simulink library "X_Plane_Communication_Library"  (R2013a)
settings: Solver=ode45  StartTime=0.0  StopTime=10.0  RelTol=1e-3
libraries: dspnetwork x4, etargetslib x4
settings Model: Creator=Adriano  LastModifiedBy=Adriano

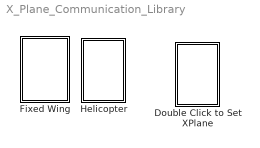
== system X_Plane_Communication_Library ==
  Double Click to Set XPlane : Subsystem
      settings: OpenFcn=selecting_parameters()
  Fixed Wing : Subsystem
  Helicopter : Subsystem

== system X_Plane_Communication_Library/Double Click to Set XPlane ==

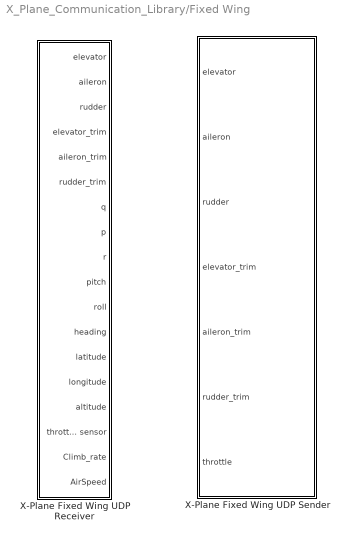
== system X_Plane_Communication_Library/Fixed Wing ==
  X-Plane Fixed Wing UDP Receiver : Subsystem  mask{ip_adress='127.0.0.1', port_number=49004}
      mask prompts: ip_adress "Local IP Adress (default: '127.0.0.1' )"; port_number "Output Port Number (defaut: '49004')"
      mask help: This block is configured to receiver data from a fixed wing aircraft on X-Plane Flight Simulator.
      mask Help: Contact adrianobittar@gmail.com
  X-Plane Fixed Wing UDP Sender : Subsystem  mask{ip_adress='127.0.0.1', port_number=49000}
      mask prompts: ip_adress "Local IP Adress (default: '127.0.0.1' )"; port_number "Output Port Number (defaut: '49000')"
      mask help: This block is configured to send data to a fixed wing aircraft on X-Plane Flight Simulator.
      mask Help: Contact adrianobittar@gmail.com

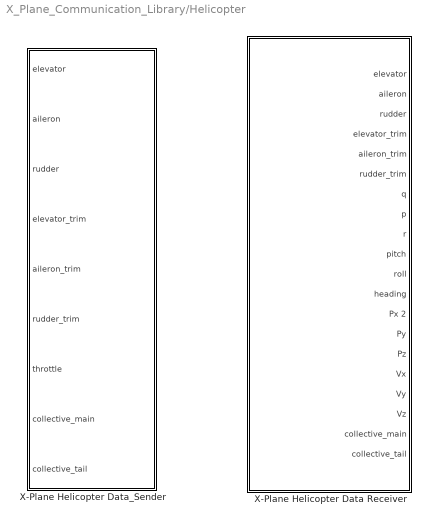
== system X_Plane_Communication_Library/Helicopter ==
  X-Plane Helicopter Data Receiver : Subsystem  AncestorBlock=DU2SRI_Heli_Sim/X-Plane Communication Blockset /X-Plane Data Receiver  mask{ip_adress='127.0.0.1', port_number=49004}
      mask prompts: ip_adress "Local IP Adress (default: '127.0.0.1')"; port_number "Input Port Number (default: '49004')"
      mask help: This block is configured to receive data to an helicopter aircraft on X-Plane Flight Simulator.
      mask Help: Contact adrianobittar@gmail.com
  X-Plane Helicopter Data_Sender : Subsystem  AncestorBlock=DU2SRI_Heli_Sim/X-Plane Communication Blockset /X-Plane Data_Sender  mask{ip_address='127.0.0.1', port_number=49000, max_col_main=12, min_col_main=0, max_col_tail=5, min_col_tail=-5}
      mask prompts: ip_address "Local IP Address (default: '127.0.0.1' )"; port_number "Output Port Number (defaut: '49000')"; max_col_main "Max Angle For Collective Main"; min_col_main "Min Angle For Collective Main"; max_col_tail "Max Angle For Collective Tail"; min_col_tail "Min Angle For Collective Tail"
      mask help: This block is configured to send data to an helicopter aircraft on X-Plane Flight Simulator.
      mask Help: contact adrianobittar@gmail.com

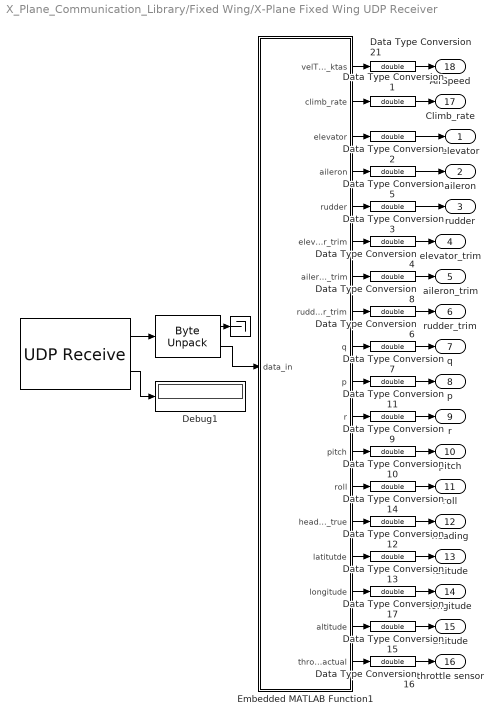
== system X_Plane_Communication_Library/Fixed Wing/X-Plane Fixed Wing UDP Receiver ==
  " " : Terminator
  "    " : dspnetwork/UDP Receive  localURL='0.0.0.0'  localPort=port_number  remoteURL=ip_adress  remotePort=-1  recvBufferSize=8192  dims=293  signalDatatype=uint8  isVarSize=off  showBlockingTime=on  blockingTime=20  sampletime=0.02  blockPlatform=WINDOWS
  "     " : etargetslib/Byte Unpack  dimensions={5,[9,8]}  datatypes={'uint8','single'}  byteAlign=1
  Data Type Conversion{1..17,21} (18 alike) : DataTypeConversion  OutDataTypeStr=double  SaturateOnIntegerOverflow=on
  "Debug1 " : Display
  Embedded MATLAB Function1 : MATLAB Function  TreatAsAtomicUnit=on
  "elevator " : Outport
  aileron : Outport  Port=2
  rudder : Outport  Port=3
  elevator_trim : Outport  Port=4
  aileron_trim : Outport  Port=5
  rudder_trim : Outport  Port=6
  q : Outport  Port=7
  p : Outport  Port=8
  r : Outport  Port=9
  pitch : Outport  Port=10
  roll : Outport  Port=11
  heading : Outport  Port=12
  latitude : Outport  Port=13
  longitude : Outport  Port=14
  altitude : Outport  Port=15
  throttle sensor : Outport  Port=16
  Climb_rate : Outport  Port=17
  AirSpeed : Outport  Port=18
  wires:
  "     "/2 -> Embedded MATLAB Function1/1(data_in)
  Data Type Conversion9/1 -> r/1
  "    "/1 -> "     "/1
  Data Type Conversion10/1 -> pitch/1
  "    "/2 -> "Debug1 "/1
  "     "/1 -> " "/1
  Embedded MATLAB Function1/1(velTrue_ktas) -> Data Type Conversion21/1
  Embedded MATLAB Function1/18(throttle_actual) -> Data Type Conversion16/1
  Embedded MATLAB Function1/17(altitude) -> Data Type Conversion15/1
  Embedded MATLAB Function1/16(longitude) -> Data Type Conversion17/1
  Embedded MATLAB Function1/15(latitutde) -> Data Type Conversion13/1
  Embedded MATLAB Function1/14(heading_true) -> Data Type Conversion12/1
  Embedded MATLAB Function1/13(roll) -> Data Type Conversion14/1
  Embedded MATLAB Function1/12(pitch) -> Data Type Conversion10/1
  Embedded MATLAB Function1/11(r) -> Data Type Conversion9/1
  Embedded MATLAB Function1/10(p) -> Data Type Conversion11/1
  Embedded MATLAB Function1/9(q) -> Data Type Conversion7/1
  Embedded MATLAB Function1/8(rudder_trim) -> Data Type Conversion6/1
  Embedded MATLAB Function1/7(aileron_trim) -> Data Type Conversion8/1
  Embedded MATLAB Function1/6(elevator_trim) -> Data Type Conversion4/1
  Embedded MATLAB Function1/5(rudder) -> Data Type Conversion3/1
  Embedded MATLAB Function1/4(aileron) -> Data Type Conversion5/1
  Embedded MATLAB Function1/3(elevator) -> Data Type Conversion2/1
  Embedded MATLAB Function1/2(climb_rate) -> Data Type Conversion1/1
  Data Type Conversion21/1 -> AirSpeed/1
  Data Type Conversion1/1 -> Climb_rate/1
  Data Type Conversion2/1 -> "elevator "/1
  Data Type Conversion5/1 -> aileron/1
  Data Type Conversion8/1 -> aileron_trim/1
  Data Type Conversion3/1 -> rudder/1
  Data Type Conversion4/1 -> elevator_trim/1
  Data Type Conversion6/1 -> rudder_trim/1
  Data Type Conversion7/1 -> q/1
  Data Type Conversion12/1 -> heading/1
  Data Type Conversion13/1 -> latitude/1
  Data Type Conversion14/1 -> roll/1
  Data Type Conversion17/1 -> longitude/1
  Data Type Conversion15/1 -> altitude/1
  Data Type Conversion16/1 -> throttle sensor/1
  Data Type Conversion11/1 -> p/1

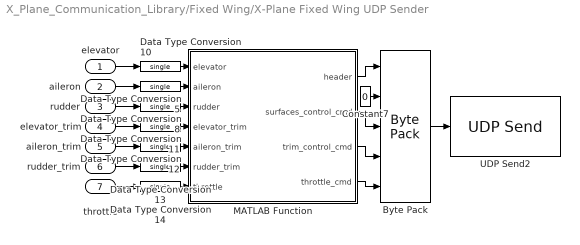
== system X_Plane_Communication_Library/Fixed Wing/X-Plane Fixed Wing UDP Sender ==
  elevator : Inport
  aileron : Inport  Port=2
  rudder : Inport  Port=3
  elevator_trim : Inport  Port=4
  aileron_trim : Inport  Port=5
  rudder_trim : Inport  Port=6
  throttle : Inport  Port=7
  Byte Pack : etargetslib/Byte Pack  datatypes={'single','uint8','single','single','single'}  byteAlign=1
  Constant7 : Constant  Value=0  OutDataTypeStr=uint8
  Data Type Conversion{5,8,10..14} (7 alike) : DataTypeConversion  OutDataTypeStr=single  SaturateOnIntegerOverflow=on
  MATLAB Function : MATLAB Function  TreatAsAtomicUnit=on
  UDP Send2 : dspnetwork/UDP Send  remoteURL=ip_adress  remotePort=port_number  localURL='255.255.255.255'  localPortSource=Automatically determine  localPort=-1  sampletime=-1  blockPlatform=HOST  separateLengthPort=0
  wires:
  rudder/1 -> Data Type Conversion8/1
  Constant7/1 -> Byte Pack/2
  Data Type Conversion8/1 -> MATLAB Function/3(rudder)
  throttle/1 -> Data Type Conversion14/1
  Data Type Conversion10/1 -> MATLAB Function/1(elevator)
  Data Type Conversion11/1 -> MATLAB Function/4(elevator_trim)
  aileron/1 -> Data Type Conversion5/1
  elevator/1 -> Data Type Conversion10/1
  MATLAB Function/4(throttle_cmd) -> Byte Pack/5
  Data Type Conversion5/1 -> MATLAB Function/2(aileron)
  Data Type Conversion14/1 -> MATLAB Function/7(throttle)
  MATLAB Function/3(trim_control_cmd) -> Byte Pack/4
  aileron_trim/1 -> Data Type Conversion12/1
  Data Type Conversion13/1 -> MATLAB Function/6(rudder_trim)
  Data Type Conversion12/1 -> MATLAB Function/5(aileron_trim)
  MATLAB Function/1(header) -> Byte Pack/1
  elevator_trim/1 -> Data Type Conversion11/1
  Byte Pack/1 -> UDP Send2/1
  MATLAB Function/2(surfaces_control_cmd) -> Byte Pack/3
  rudder_trim/1 -> Data Type Conversion13/1

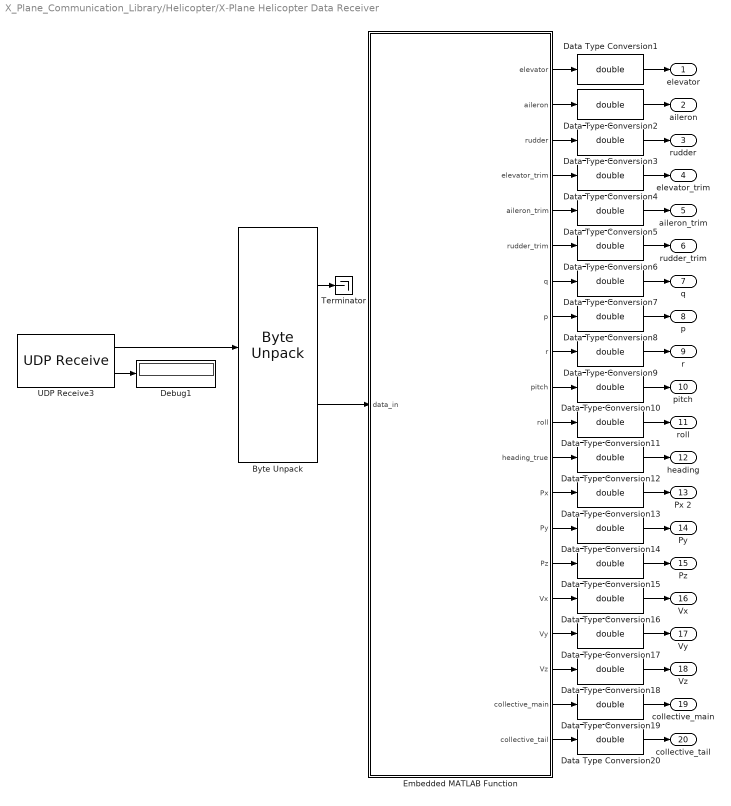
== system X_Plane_Communication_Library/Helicopter/X-Plane Helicopter Data Receiver ==
  Byte Unpack : etargetslib/Byte Unpack  dimensions={5,[9,6]}  datatypes={'uint8','single'}  byteAlign=1
  Data Type Conversion{1..20} (20 alike) : DataTypeConversion  OutDataTypeStr=double  SaturateOnIntegerOverflow=on
  "Debug1 " : Display
  Embedded MATLAB Function : MATLAB Function  TreatAsAtomicUnit=on
  Terminator : Terminator
  UDP Receive3 : dspnetwork/UDP Receive  localURL='0.0.0.0'  localPort=port_number  remoteURL=ip_adress  remotePort=-1  recvBufferSize=8192  dims=221  signalDatatype=uint8  isVarSize=off  showBlockingTime=on  blockingTime=20  sampletime=0  blockPlatform=WINDOWS
  "elevator " : Outport
  aileron : Outport  Port=2
  rudder : Outport  Port=3
  elevator_trim : Outport  Port=4
  aileron_trim : Outport  Port=5
  rudder_trim : Outport  Port=6
  q : Outport  Port=7
  p : Outport  Port=8
  r : Outport  Port=9
  pitch : Outport  Port=10
  roll : Outport  Port=11
  heading : Outport  Port=12
  Px 2 : Outport  Port=13
  Py : Outport  Port=14
  Pz : Outport  Port=15
  Vx : Outport  Port=16
  Vy : Outport  Port=17
  Vz : Outport  Port=18
  collective_main : Outport  Port=19
  collective_tail : Outport  Port=20
  wires:
  Embedded MATLAB Function/10(pitch) -> Data Type Conversion10/1
  Data Type Conversion8/1 -> p/1
  Data Type Conversion13/1 -> Px 2/1
  Data Type Conversion1/1 -> "elevator "/1
  Byte Unpack/1 -> Terminator/1
  UDP Receive3/2 -> "Debug1 "/1
  Data Type Conversion4/1 -> elevator_trim/1
  Embedded MATLAB Function/8(p) -> Data Type Conversion8/1
  Data Type Conversion12/1 -> heading/1
  Embedded MATLAB Function/11(roll) -> Data Type Conversion11/1
  Embedded MATLAB Function/1(elevator) -> Data Type Conversion1/1
  Data Type Conversion10/1 -> pitch/1
  Embedded MATLAB Function/3(rudder) -> Data Type Conversion3/1
  Data Type Conversion2/1 -> aileron/1
  Data Type Conversion6/1 -> rudder_trim/1
  UDP Receive3/1 -> Byte Unpack/1
  Data Type Conversion9/1 -> r/1
  Data Type Conversion11/1 -> roll/1
  Embedded MATLAB Function/7(q) -> Data Type Conversion7/1
  Embedded MATLAB Function/18(Vz) -> Data Type Conversion18/1
  Data Type Conversion18/1 -> Vz/1
  Data Type Conversion5/1 -> aileron_trim/1
  Data Type Conversion15/1 -> Pz/1
  Data Type Conversion19/1 -> collective_main/1
  Embedded MATLAB Function/14(Py) -> Data Type Conversion14/1
  Embedded MATLAB Function/5(aileron_trim) -> Data Type Conversion5/1
  Embedded MATLAB Function/19(collective_main) -> Data Type Conversion19/1
  Embedded MATLAB Function/6(rudder_trim) -> Data Type Conversion6/1
  Embedded MATLAB Function/20(collective_tail) -> Data Type Conversion20/1
  Data Type Conversion16/1 -> Vx/1
  Embedded MATLAB Function/12(heading_true) -> Data Type Conversion12/1
  Embedded MATLAB Function/13(Px) -> Data Type Conversion13/1
  Data Type Conversion17/1 -> Vy/1
  Embedded MATLAB Function/4(elevator_trim) -> Data Type Conversion4/1
  Data Type Conversion14/1 -> Py/1
  Embedded MATLAB Function/17(Vy) -> Data Type Conversion17/1
  Embedded MATLAB Function/2(aileron) -> Data Type Conversion2/1
  Embedded MATLAB Function/16(Vx) -> Data Type Conversion16/1
  Data Type Conversion3/1 -> rudder/1
  Embedded MATLAB Function/15(Pz) -> Data Type Conversion15/1
  Embedded MATLAB Function/9(r) -> Data Type Conversion9/1
  Data Type Conversion7/1 -> q/1
  Data Type Conversion20/1 -> collective_tail/1
  Byte Unpack/2 -> Embedded MATLAB Function/1(data_in)

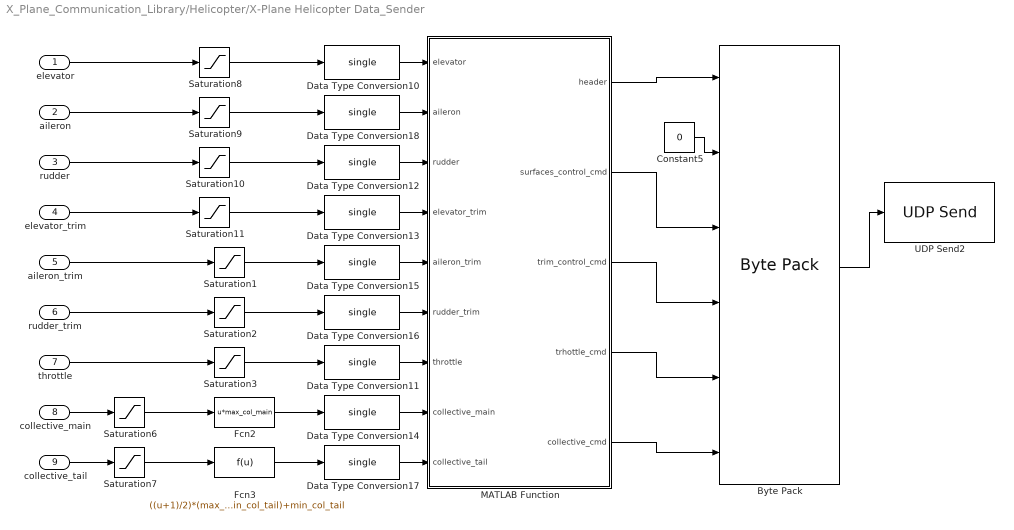
== system X_Plane_Communication_Library/Helicopter/X-Plane Helicopter Data_Sender ==
  elevator : Inport
  aileron : Inport  Port=2
  rudder : Inport  Port=3
  elevator_trim : Inport  Port=4
  aileron_trim : Inport  Port=5
  rudder_trim : Inport  Port=6
  throttle : Inport  Port=7
  collective_main : Inport  Port=8
  collective_tail : Inport  Port=9
  Byte Pack : etargetslib/Byte Pack  datatypes={'single','uint8','single','single','single','single'}  byteAlign=1
  Constant5 : Constant  Value=0  OutDataTypeStr=uint8
  Data Type Conversion{10..18} (9 alike) : DataTypeConversion  OutDataTypeStr=single  SaturateOnIntegerOverflow=on
  Fcn2 : Fcn  Expr=u*max_col_main
  Fcn3 : Fcn  Expr=((u+1)/2)*(max_col_tail-min_col_tail)+min_col_tail
  MATLAB Function : MATLAB Function  TreatAsAtomicUnit=on
  Saturation{1..3,6..11} (9 alike) : Saturate  UpperLimit=+1  LowerLimit=-1
  UDP Send2 : dspnetwork/UDP Send  remoteURL=ip_address  remotePort=port_number  localURL='255.255.255.255'  localPortSource=Automatically determine  localPort=-1  sampletime=-1  blockPlatform=HOST  separateLengthPort=0
  wires:
  Saturation8/1 -> Data Type Conversion10/1
  Data Type Conversion18/1 -> MATLAB Function/2(aileron)
  Constant5/1 -> Byte Pack/2
  MATLAB Function/5(collective_cmd) -> Byte Pack/6
  MATLAB Function/4(trhottle_cmd) -> Byte Pack/5
  MATLAB Function/3(trim_control_cmd) -> Byte Pack/4
  MATLAB Function/2(surfaces_control_cmd) -> Byte Pack/3
  MATLAB Function/1(header) -> Byte Pack/1
  Byte Pack/1 -> UDP Send2/1
  Data Type Conversion17/1 -> MATLAB Function/9(collective_tail)
  Data Type Conversion14/1 -> MATLAB Function/8(collective_main)
  Data Type Conversion11/1 -> MATLAB Function/7(throttle)
  Data Type Conversion16/1 -> MATLAB Function/6(rudder_trim)
  Data Type Conversion15/1 -> MATLAB Function/5(aileron_trim)
  Data Type Conversion13/1 -> MATLAB Function/4(elevator_trim)
  Data Type Conversion12/1 -> MATLAB Function/3(rudder)
  Data Type Conversion10/1 -> MATLAB Function/1(elevator)
  Saturation10/1 -> Data Type Conversion12/1
  Saturation11/1 -> Data Type Conversion13/1
  Saturation9/1 -> Data Type Conversion18/1
  Saturation7/1 -> Fcn3/1
  Saturation6/1 -> Fcn2/1
  collective_main/1 -> Saturation6/1
  collective_tail/1 -> Saturation7/1
  Saturation3/1 -> Data Type Conversion11/1
  elevator_trim/1 -> Saturation11/1
  Saturation1/1 -> Data Type Conversion15/1
  aileron/1 -> Saturation9/1
  Saturation2/1 -> Data Type Conversion16/1
  elevator/1 -> Saturation8/1
  Fcn2/1 -> Data Type Conversion14/1
  rudder/1 -> Saturation10/1
  aileron_trim/1 -> Saturation1/1
  rudder_trim/1 -> Saturation2/1
  throttle/1 -> Saturation3/1
  Fcn3/1 -> Data Type Conversion17/1

== matlab function X_Plane_Communication_Library/Fixed Wing/X-Plane Fixed Wing UDP Receiver/Embedded MATLAB Function1 ==
  data: velTrue_ktas output; climb_rate output; data_in input; elevator output; aileron output; rudder output; elevator_trim output; aileron_trim output; rudder_trim output; q output; p output; r output; pitch output; roll output; heading_true output; latitutde output; longitude output; altitude output; throttle_actual output
function [velTrue_ktas, climb_rate,elevator, aileron, rudder, elevator_trim, aileron_trim, rudder_trim, q,p,r, pitch, roll, heading_true, latitutde, longitude, altitude, throttle_actual]   = fcn(data_in)
% This block supports the Embedded MATLAB subset.
% See the help menu for details. 


velTrue_ktas = data_in(4,1);

climb_rate = data_in(4,2);

elevator = data_in(2,3);
aileron = data_in(3,3);
rudder= data_in(4,3);


elevator_trim= data_in(2,4);
aileron_trim= data_in(3,4);
rudder_trim= data_in(4,4);

q= data_in(2,5);
p= data_in(3,5);
r= data_in(4,5);

pitch= data_in(2,6);
roll= data_in(3,6);
heading_true= data_in(4,6);

latitutde= data_in(2,7);
longitude= data_in(3,7);
altitude= data_in(4,7);


throttle_actual = data_in(2,8);

== matlab function X_Plane_Communication_Library/Helicopter/X-Plane Helicopter Data_Sender/MATLAB Function ==
  data: elevator input single size=1; aileron input; rudder input; elevator_trim input; aileron_trim input; rudder_trim input; throttle input; collective_main input; collective_tail input; header output single size=1; surfaces_control_cmd output single size=[1 18]; trim_control_cmd output single size=[1 18]; trhottle_cmd output single size=[1 9]; collective_cmd output single size=[1 9]
function [header, surfaces_control_cmd,trim_control_cmd,trhottle_cmd,collective_cmd]  = fcn(elevator, aileron, rudder, elevator_trim, aileron_trim, rudder_trim, throttle, collective_main, collective_tail)
% This block supports the Embedded MATLAB subset.
% See the help menu for details. 

header = typecast(uint8([uint8(68) uint8(65) uint8(84) uint8(65)]), 'single');




No_Comand = single(-999);

Surface_header = typecast(uint8([uint8(8) uint8(0) uint8(0) uint8(0)]), 'single');

surfaces_control_cmd = [Surface_header elevator aileron rudder No_Comand No_Comand No_Comand No_Comand No_Comand Surface_header No_Comand No_Comand No_Comand No_Comand No_Comand No_Comand No_Comand No_Comand];

Trim_header = typecast(uint8([uint8(13) uint8(0) uint8(0) uint8(0)]), 'single');


trim_control_cmd = [ Trim_header elevator_trim aileron_trim rudder_trim No_Comand No_Comand No_Comand No_Comand No_Comand Trim_header No_Comand No_Comand No_Comand No_Comand No_Comand No_Comand No_Comand No_Comand];

Throttle_header = typecast(uint8([uint8(25) uint8(0) uint8(0) uint8(0)]), 'single');
trhottle_cmd = [Throttle_header throttle No_Comand No_Comand No_Comand No_Comand No_Comand No_Comand No_Comand];

Collective_header = typecast(uint8([uint8(39) uint8(0) uint8(0) uint8(0)]), 'single');

collective_cmd = [ Collective_header collective_main collective_tail No_Comand No_Comand No_Comand No_Comand No_Comand No_Comand];
%data_out = [surfaces_control_cmd trim_control_cmd trhottle_cmd collective_cmd];


% Actuadors_Out[0] = 68;
% Actuadors_Out[1] = 65;
% Actuadors_Out[2] = 84;
% Actuadors_Out[3] = 65;
% Actuadors_Out[4] = 48;//26;
% aileron = data_in(3,1);
% rudder= data_in(4,1);
% 
% 
% elevator_trim= data_in(2,2);
% aileron_trim= data_in(3,2);
% rudder_trim= data_in(4,2);
% 
% q= data_in(2,3);
% p= data_in(3,3);
% r= data_in(4,3);
% 
% pitch= data_in(2,4);
% roll= data_in(3,4);
% heading_true= data_in(4,4);
% 
% Px= data_in(2,5);
% Py= data_in(3,5);
% Pz= data_in(4,5);
% Vx= data_in(5,5);
% Vy= data_in(6,5);
% Vz= data_in(7,5);
% 
% collective_main= data_in(2,6);
% collective_tail= data_in(3,6);

== matlab function X_Plane_Communication_Library/Fixed Wing/X-Plane Fixed Wing UDP Sender/MATLAB Function ==
  data: elevator input single size=1; aileron input; rudder input; elevator_trim input; aileron_trim input; rudder_trim input; throttle input; header output single size=1; surfaces_control_cmd output single size=[1 18]; trim_control_cmd output single size=[1 18]; throttle_cmd output size=[1 18]
function [header, surfaces_control_cmd,trim_control_cmd, throttle_cmd]  = fcn(elevator, aileron, rudder, elevator_trim, aileron_trim, rudder_trim, throttle)
% This block supports the Embedded MATLAB subset.
% See the help menu for details. 

header = typecast(uint8([uint8(68) uint8(65) uint8(84) uint8(65)]), 'single');



No_Comand = single(-999);

Surface_header = typecast(uint8([uint8(8) uint8(0) uint8(0) uint8(0)]), 'single');

surfaces_control_cmd = [Surface_header elevator aileron rudder No_Comand No_Comand No_Comand No_Comand No_Comand Surface_header No_Comand No_Comand No_Comand No_Comand No_Comand No_Comand No_Comand No_Comand];

Trim_header = typecast(uint8([uint8(13) uint8(0) uint8(0) uint8(0)]), 'single');


trim_control_cmd = [ Trim_header elevator_trim aileron_trim rudder_trim No_Comand No_Comand No_Comand No_Comand No_Comand Trim_header No_Comand No_Comand No_Comand No_Comand No_Comand No_Comand No_Comand No_Comand];

Throttle_header = typecast(uint8([uint8(25) uint8(0) uint8(0) uint8(0)]), 'single');
throttle_cmd = [Throttle_header throttle No_Comand No_Comand No_Comand No_Comand No_Comand No_Comand No_Comand Throttle_header No_Comand No_Comand No_Comand No_Comand No_Comand No_Comand No_Comand No_Comand];




% Actuadors_Out[0] = 68;
% Actuadors_Out[1] = 65;
% Actuadors_Out[2] = 84;
% Actuadors_Out[3] = 65;
% Actuadors_Out[4] = 48;//26;
% aileron = data_in(3,1);
% rudder= data_in(4,1);
% 
% 
% elevator_trim= data_in(2,2);
% aileron_trim= data_in(3,2);
% rudder_trim= data_in(4,2);
% 
% q= data_in(2,3);
% p= data_in(3,3);
% r= data_in(4,3);
% 
% pitch= data_in(2,4);
% roll= data_in(3,4);
% heading_true= data_in(4,4);
% 
% Px= data_in(2,5);
% Py= data_in(3,5);
% Pz= data_in(4,5);
% Vx= data_in(5,5);
% Vy= data_in(6,5);
% Vz= data_in(7,5);
% 
% collective_main= data_in(2,6);
% collective_tail= data_in(3,6);

== matlab function X_Plane_Communication_Library/Helicopter/X-Plane Helicopter Data Receiver/Embedded MATLAB Function ==
  data: data_in input; elevator output; aileron output; rudder output; elevator_trim output; aileron_trim output; rudder_trim output; q output; p output; r output; pitch output; roll output; heading_true output; Px output; Py output; Pz output; Vx output; Vy output; Vz output; collective_main output; collective_tail output
function [elevator, aileron, rudder, elevator_trim, aileron_trim, rudder_trim, q,p,r, pitch, roll, heading_true, Px, Py, Pz, Vx, Vy, Vz, collective_main, collective_tail]   = fcn(data_in)
% This block supports the Embedded MATLAB subset.
% See the help menu for details. 

elevator = data_in(2,1);
aileron = data_in(3,1);
rudder= data_in(4,1);


elevator_trim= data_in(2,2);
aileron_trim= data_in(3,2);
rudder_trim= data_in(4,2);

q= data_in(2,3);
p= data_in(3,3);
r= data_in(4,3);

pitch= data_in(2,4);
roll= data_in(3,4);
heading_true= data_in(4,4);

Px= data_in(2,5);
Py= data_in(3,5);
Pz= data_in(4,5);
Vx= data_in(5,5);
Vy= data_in(6,5);
Vz= data_in(7,5);

collective_main= data_in(2,6);
collective_tail= data_in(3,6);
